simulink model "pendulum_3a1_ez"  (R2018b)
settings: Solver=VariableStepAuto  StartTime=0.0  StopTime=500  RelTol=1e-3
values from neighbouring files (symbols this model uses):
  A = [0 0 1 0 ... (first row only)    [pendulum_version1.m]
  B = [0;0;Km*Kg/(Cart_m*Rm*motor_radius);-Km*Kg/(Cart_m*Rm*motor_radius*Rod_l)]    [pendulum_version1.m]
  C_ez = eye(4)    [pendulum_version1.m]
  CC = [0.456/4.41 0; 0 90/6.328]    [pendulum_version1.m]
  D_ez = zeros(4,1)    [pendulum_version1.m]
  K = lqr(A,B,Q1,R)    [pendulum_version1.m]
settings Model: Creator=paul-emileverleye  LastModifiedBy=Kyle
settings DebuggingCC: LibraryContextMissingDiagnostic=none
settings SFSimCC: SimUseLocalCustomCode=off
settings RTWCC: RTWUseLocalCustomCode=off

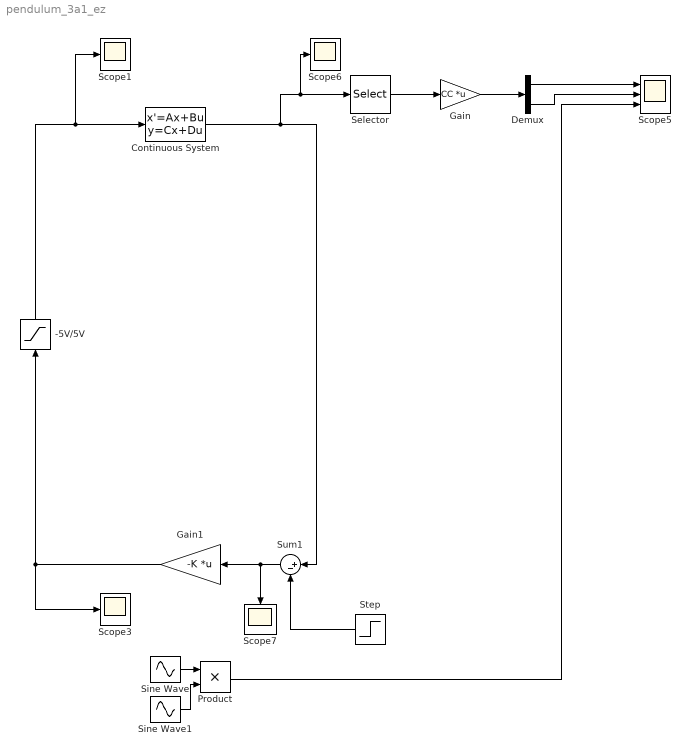
== system pendulum_3a1_ez ==
  -5V/5V : Saturate  UpperLimit=5  LowerLimit=-5
  Continuous System : StateSpace  A=A  B=B  C=C_ez  D=D_ez  InitialCondition=0
  Demux : Demux  Outputs=2
  Gain : Gain  Gain=CC  Multiplication=Matrix(K*u)
  Gain1 : Gain  Gain=-K  Multiplication=Matrix(K*u)
  Product : Product
  Scope{1,3,6..7} (4 alike) : Scope
  Scope5 : Scope  NumInputPorts=3
  Selector : Selector  InputPortWidth=4  IndexOptions=Index vector (dialog)  Indices=[1 2]  OutputSizes=1
  Sine Wave : Sin  Frequency=0.1  SampleTime=0
  Sine Wave1 : Sin  Frequency=0.01  SampleTime=0
  Step : Step  After=0.1  SampleTime=0
  Sum1 : Sum  Inputs=|+-
  wires:
  Gain1/1 -> Scope3/1, -5V/5V/1
  -5V/5V/1 -> Continuous System/1, Scope1/1
  Demux/1 -> Scope5/1
  Gain/1 -> Demux/1
  Demux/2 -> Scope5/2
  Sum1/1 -> Scope7/1, Gain1/1
  Continuous System/1 -> Sum1/1, Scope6/1, Selector/1
  Sine Wave/1 -> Product/1
  Sine Wave1/1 -> Product/2
  Product/1 -> Scope5/3
  Selector/1 -> Gain/1
  Step/1 -> Sum1/2
